simulink model "Climb"  (R2024a)
settings: Solver=VariableStepAuto  StartTime=0.0  StopTime=55  RelTol=1e-3
values from neighbouring files (symbols this model uses):
  beta0 = 1    [data.m]
  Map_CD = ReshapeMatrix(data0,data4,data8,flag_CD)    [data.m]
  Map_CL = ReshapeMatrix(data0,data4,data8,flag_CL)    [data.m]
undefined symbols (not defined in the file or in its folder): FullWeight, Sc
libraries: aerolibatmos2 x1, simulink x1
settings Model: Creator=10335  LastModifiedBy=10335

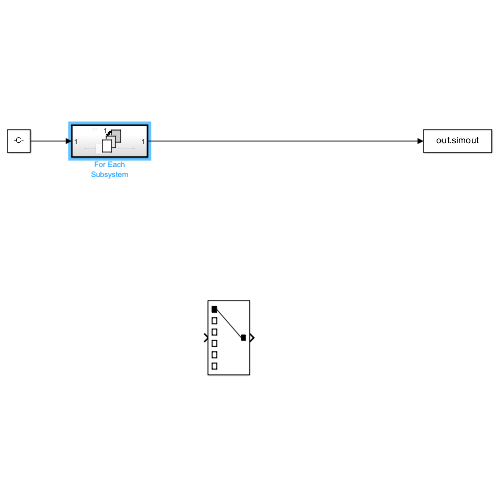
[thumbnail: Simulink's stored preview of the top-level diagram]
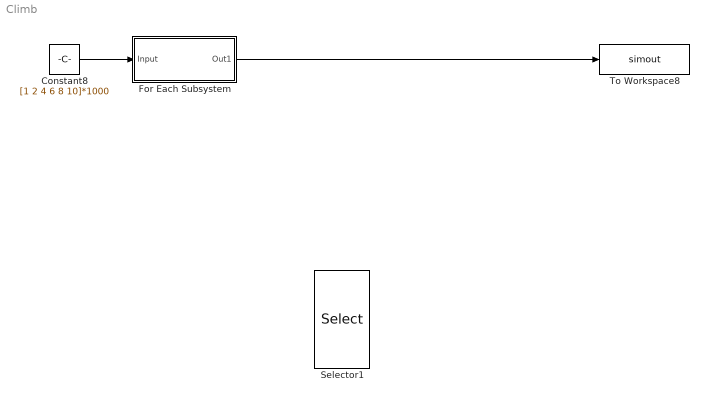
== system Climb ==
  Constant8 : Constant  Value=[1 2 4 6 8 10]*1000
  For Each Subsystem : Subsystem  TreatAsAtomicUnit=on
  Selector1 : Selector  InputPortWidth=6  IndexOptions=Index vector (dialog)  Indices=[1]  OutputSizes=1
  To Workspace8 : ToWorkspace  VariableName=simout  SaveFormat=Timeseries  SampleTime=-1
  wires:
  Constant8/1 -> For Each Subsystem/1(Input)
  For Each Subsystem/1(Out1) -> To Workspace8/1

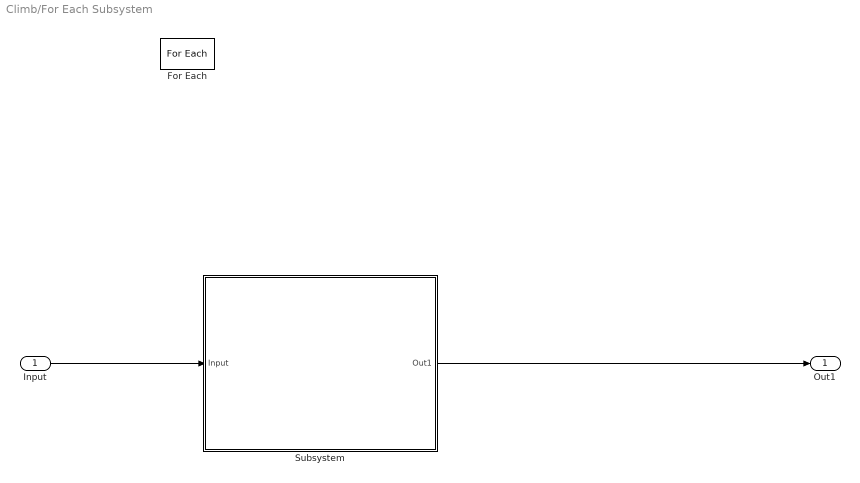
== system Climb/For Each Subsystem ==
  Input : Inport  Partition=on  PartitionDimension=2  PartitionWidth=1  PartitionOffset=0
  For Each : ForEach  DisableCoverage=on
  Subsystem : Subsystem
  Out1 : Outport  ConcatenationDimension=1
  wires:
  Input/1 -> Subsystem/1(Input)
  Subsystem/1(Out1) -> Out1/1

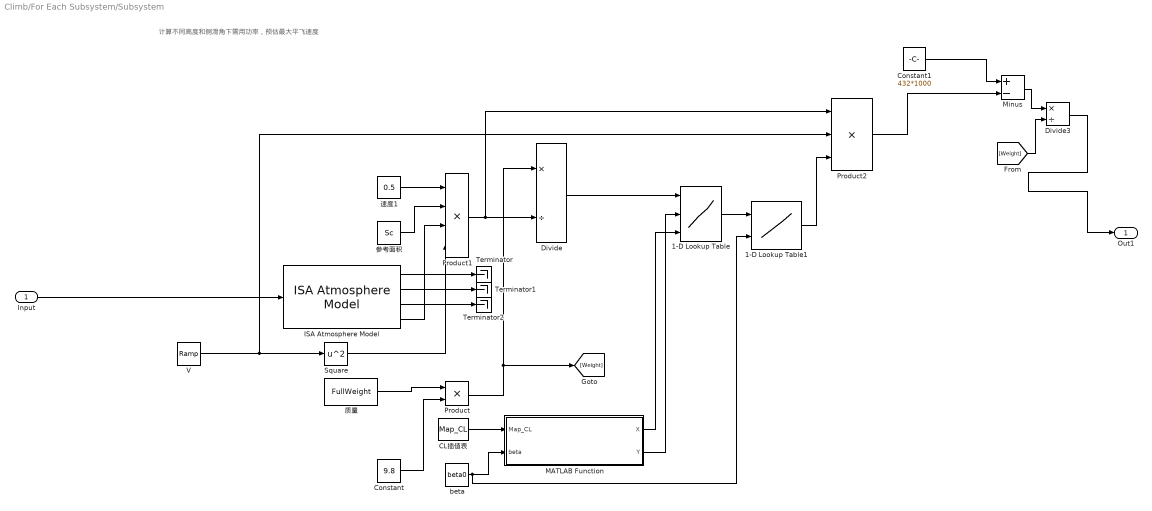
== system Climb/For Each Subsystem/Subsystem ==
  note: 计算不同高度和侧滑角下需用功率，预估最大平飞速度
  Input : Inport
  1-D Lookup Table : Lookup_n-D  NumberOfTableDimensions=1  BreakpointsForDimension1Source=Input port  BreakpointsForDimension1=[-5:5]  TableSource=Input port  Table=tanh([-5:5])  InternalRulePriority=Speed  RndMeth=Simplest
      settings: InputPortMap=u0,p221,p5
  1-D Lookup Table1 : Lookup_n-D  BreakpointsForDimension1=[0 4 8]  BreakpointsForDimension2=[0 5 10 15 20 25]  Table=Map_CD  InternalRulePriority=Speed  RndMeth=Simplest
      settings: InputPortMap=u0,u1
  CL插值表 : Constant  Value=Map_CL
  Constant : Constant  Value=9.8
  Constant1 : Constant  Value=432*1000
  Divide : Product  Inputs=*/
  Divide3 : Product  Inputs=*/
  ISA Atmosphere Model : aerolibatmos2/ISA Atmosphere Model  useExtended=off  action=Warning  custom=off  viscosityOut=off  g=9.80665  gamma=1.4  R=287.0531  L=0.0065  h_trop=11000  h_strat=20000  rho0=1.225  P0=101325  T0=288.15  h0=0  S=110.4  Tref=273.15  muref=1.716e-5
  MATLAB Function : MATLAB Function  TreatAsAtomicUnit=on
  Minus : Sum  Inputs=+-
  Product : Product
  Product1 : Product  Inputs=4
  Product2 : Product  Inputs=3
  Square : Math  Operator=square
  Terminator : Terminator
  Terminator1 : Terminator
  Terminator2 : Terminator
  V : simulink/Sources/Ramp  slope=1  start=0  InitialOutput=45
  beta : Constant  Value=beta0
  参考面积 : Constant  Value=Sc
  质量 : Constant  Value=FullWeight
  速度1 : Constant  Value=0.5
  Out1 : Outport
  wires:
  Divide3/1 -> Out1/1
  V/1 -> Product2/2, Square/1
  Divide/1 -> 1-D Lookup Table/1
  Product2/1 -> Minus/2
  Constant/1 -> Product/2
  beta/1 -> 1-D Lookup Table1/2, MATLAB Function/2(beta)
  Product1/1 -> Product2/1, Divide/2
  速度1/1 -> Product1/1
  Square/1 -> Product1/4
  Minus/1 -> Divide3/1
  质量/1 -> Product/1
  1-D Lookup Table/1 -> 1-D Lookup Table1/1
  MATLAB Function/1(X) -> 1-D Lookup Table/3
  ISA Atmosphere Model/4 -> Product1/3
  Input/1 -> ISA Atmosphere Model/1
  CL插值表/1 -> MATLAB Function/1(Map_CL)
  Product/1 -> Divide/1, [Weight]
  1-D Lookup Table1/1 -> Product2/3
  MATLAB Function/2(Y) -> 1-D Lookup Table/2
  Constant1/1 -> Minus/1
  ISA Atmosphere Model/3 -> Terminator2/1
  参考面积/1 -> Product1/2
  ISA Atmosphere Model/1 -> Terminator/1
  [Weight] -> Divide3/2
  ISA Atmosphere Model/2 -> Terminator1/1

== matlab function Climb/For Each Subsystem/Subsystem/MATLAB Function ==
  data: Map_CL input; X output; beta input; Y output

function [X,Y]=InvMatrix(Map_CL,beta)
X=Map_CL(1:3,beta)';
Y=[0 4 8];
